simulink model "inverter_control"  (Simulink 8.5)
settings: Solver=ode23tb  StartTime=0.0  StopTime=0.1  RelTol=1e-4
values from neighbouring files (symbols this model uses):
  f_grid = 50    [inverter_settings.m]
  Kp = 2    [inverter_settings.m]
  L_f = 2e-3    (= 0.002)    [inverter_settings.m]
  R_f = 10e-3    (= 0.01)    [inverter_settings.m]
  Ti = 10e-3    (= 0.01)    [inverter_settings.m]
  V_dc = 700    [inverter_settings.m]
  V_grid = 230    [inverter_settings.m]
  wc = 1/0.05e-3    (= 20000)    [inverter_settings.m]
undefined symbols (not defined in the file or in its folder): j
libraries: powerlib x28, powerlib_meascontrol x3
settings Model: Creator=Pierre  LastModifiedBy=Pierre
settings DataIOCC: SignalLoggingSaveFormat=Dataset
settings OptimizationCC: ExpressionDepthLimit=128
settings DebuggingCC: UnderspecifiedInitializationDetection=Simplified  MergeDetectMultiDrivingBlocksExec=error  FcnCallInpInsideContextMsg=EnableAllAsError  StateNameClashWarn=none
settings GRTTargetCC: CombineOutputUpdateFcns=on  GRTInterface=off

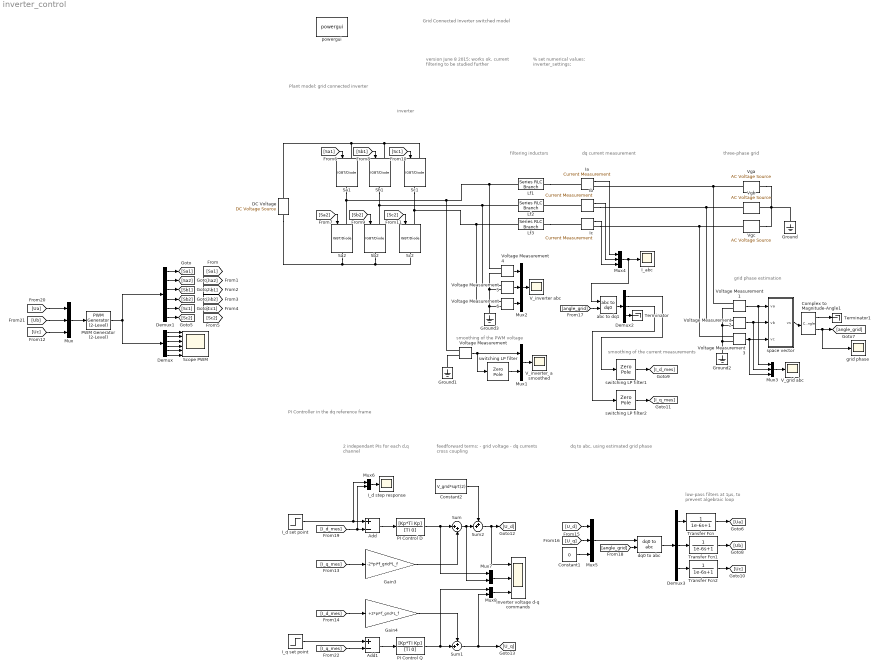
== system inverter_control ==
  note: smoothing of the current measurements
  note: feedforward terms:
      | - grid voltage
      | - dq currents cross coupling
  note: PI Controller
      | in the dq reference frame
  note: % set numerical values:
      | inverter_settings;
  note: version June 8 2015: works ok.
      | current filtering to be studied further
  note: Grid Connected Inverter
      | switched model
  note: 2 independant PIs
      | for each d,q channel
  note: dq to abc,
      | using estimated grid phase
  note: low-pass filters at 1µs,
      | to prevent algebraic loop
  note: inverter
  note: Plant model: grid connected inverter
  note: filtering inductors
  note: three-phase grid
  note: dq current measurement
  note: grid phase estimation
  note: smoothing of the PWM voltage
  Add : Sum  Inputs=+-
  Add1 : Sum  Inputs=+-
  Complex to Magnitude-Angle1 : ComplexToMagnitudeAngle
  Constant1 : Constant  Value=0
  Constant2 : Constant  Value=V_grid*sqrt(2)
  DC Voltage : powerlib/Electrical Sources/DC Voltage Source  Amplitude=V_dc  Measurements=None
  Demux : Demux  Outputs=6
  Demux1 : Demux  Outputs=6
  Demux2 : Demux  Outputs=3
  Demux3 : Demux  Outputs=3
  Gain3 : Gain  Gain=-2*pi*f_grid*L_f
  Gain4 : Gain  Gain=+2*pi*f_grid*L_f
  Ground{,1..3} (4 alike) : powerlib/Elements/Ground  LConnTagsString=a
  I_abc : Scope
      settings: TimeRange=2  YMin=0  YMax=12  SaveName=ScopeData4
  I_d set point : Step  Time=0.03  After=10  SampleTime=0
  I_d step response : Scope
      settings: TimeRange=2  YMin=-15  YMax=15  SaveName=ScopeData7
  I_q set point : Step  Time=0.01  After=0  SampleTime=0
  Ia : powerlib/Measurements/Current Measurement  PhasorSimulation=off  OutputType=Complex  PSBequivalent=0
  Ib : powerlib/Measurements/Current Measurement  PhasorSimulation=off  OutputType=Complex  PSBequivalent=0
  Ic : powerlib/Measurements/Current Measurement  PhasorSimulation=off  OutputType=Complex  PSBequivalent=0
  Inverter voltage d-q commands : Scope  NumInputPorts=3
      settings: TimeRange=2  YMin=0~-5~-5  YMax=12~5~5  SaveName=ScopeData6
  Lf1 : powerlib/Elements/Series RLC Branch  LConnTagsString=__new0  RConnTagsString=__new0  BranchType=RL  Resistance=R_f  Inductance=L_f  SetiL0=off  InitialCurrent=0  Capacitance=1e-6  Setx0=off  InitialVoltage=0  Measurements=None
  Lf2 : powerlib/Elements/Series RLC Branch  LConnTagsString=__new0  RConnTagsString=__new0  BranchType=RL  Resistance=R_f  Inductance=L_f  SetiL0=off  InitialCurrent=0  Capacitance=1e-6  Setx0=off  InitialVoltage=0  Measurements=None
  Lf3 : powerlib/Elements/Series RLC Branch  LConnTagsString=__new0  RConnTagsString=__new0  BranchType=RL  Resistance=R_f  Inductance=L_f  SetiL0=off  InitialCurrent=0  Capacitance=1e-6  Setx0=off  InitialVoltage=0  Measurements=None
  Mux{,2..5} (5 alike) : Mux  Inputs=3
  Mux{1,6..8} (4 alike) : Mux  Inputs=2
  PI Control D : TransferFcn  Numerator=[Kp*Ti Kp]  Denominator=[Ti 0]
  PI Control Q : TransferFcn  Numerator=[Kp*Ti Kp]  Denominator=[Ti 0]
  PWM Generator (2-Level) : powerlib_meascontrol/Pulse & Signal Generators/PWM Generator (2-Level)  ModulatorType=Three-phase bridge (6 pulses)  ModulatorMode=Unsynchronized  Fc=f_switch  Pc=90  nF=27  MinMax=[ -V_dc/2 V_dc/2 ]  SamplingTechnique=Symmetrical regular (single edge)  ModulatingSignals=off  m=0.8  Freq=60  Phase=0  Ts=0  ShowCarrierOutport=off
  Sa1 : powerlib/Power Electronics/IGBT//Diode  Ron=1e-3  Rs=1e5  Cs=inf  Measurements=off
  Sa2 : powerlib/Power Electronics/IGBT//Diode  Ron=1e-3  Rs=1e5  Cs=inf  Measurements=off
  Sb1 : powerlib/Power Electronics/IGBT//Diode  Ron=1e-3  Rs=1e5  Cs=inf  Measurements=off
  Sb2 : powerlib/Power Electronics/IGBT//Diode  Ron=1e-3  Rs=1e5  Cs=inf  Measurements=off
  Sc1 : powerlib/Power Electronics/IGBT//Diode  Ron=1e-3  Rs=1e5  Cs=inf  Measurements=off
  Sc2 : powerlib/Power Electronics/IGBT//Diode  Ron=1e-3  Rs=1e5  Cs=inf  Measurements=off
  Scope PWM : Scope  NumInputPorts=6
      settings: YMin=-5~-5~-5~-5~-5~-5  YMax=5~5~5~5~5~5
  Sum : Sum  Inputs=|++
  Sum1 : Sum  Inputs=++|
  Sum2 : Sum  Inputs=++|
  Terminator : Terminator
  Terminator1 : Terminator
  Transfer Fcn : TransferFcn  Denominator=[1e-6 1]
  Transfer Fcn1 : TransferFcn  Denominator=[1e-6 1]
  Transfer Fcn2 : TransferFcn  Denominator=[1e-6 1]
  V_grid abc : Scope
      settings: TimeRange=2  YMin=0  YMax=12  SaveName=ScopeData2
  V_inverter abc : Scope
      settings: TimeRange=2  YMin=0  YMax=12  SaveName=ScopeData5
  V_inverter_a smoothed : Scope
      settings: TimeRange=0.01780812410426348  YMin=-450  YMax=450
  Vga : powerlib/Electrical Sources/AC Voltage Source  Amplitude=V_grid*sqrt(2)  Phase=0  Frequency=f_grid  SampleTime=0  Measurements=None
  Vgb : powerlib/Electrical Sources/AC Voltage Source  Amplitude=V_grid*sqrt(2)  Phase=-120  Frequency=f_grid  SampleTime=0  Measurements=None
  Vgc : powerlib/Electrical Sources/AC Voltage Source  Amplitude=V_grid*sqrt(2)  Phase=-240  Frequency=f_grid  SampleTime=0  Measurements=None
  Voltage Measurement{,1..6} (7 alike) : powerlib/Measurements/Voltage Measurement  PhasorSimulation=off  OutputType=Complex  PSBequivalent=0
  abc to dq1 : powerlib_meascontrol/Transformations/abc to dq0  Alignment=Aligned with phase A axis
  dq0 to abc : powerlib_meascontrol/Transformations/dq0 to abc  Alignment=Aligned with phase A axis
  grid phase : Scope
      settings: TimeRange=2  YMin=0  YMax=12  SaveName=ScopeData3
  powergui : powerlib/powergui  Priority=1  SimulationMode=Continuous  SolverType=Tustin/Backward Euler (TBE)  SampleTime=50e-6  frequency=60  SPID=off  DisableSnubberDevices=on  DisableRonSwitches=on  DisableVfSwitches=on  SwTol=0  DisplayEquations=off  Interpol=off  methode=off  Ts=100  FunctionMessages=off  echomessages=off  HookPort=off  EnableUseOfTLC=off  x0status=blocks  frequencyindice=50  Pbase=100e6  ErrMax=1e-4  Iterations=50  UnitsV=kV  UnitsW=MW  buscounter=0  RestoreLinks=warning  ResistiveCurrentMeasurement=off  Frange=[0:2:500]  Ylog=off  Xlog=on  ShowGrid=off  save=off  variable=ZData  structure=0  ZoomFFT=off  StartTime=0.0  cycles=1  DisplayStyle=1  fundamental=60  FreqAxis=off  MaxFrequency=1000  frequencyindicesteady=1  RmsSteady=1  display=off
  space vector : Subsystem
  switching LP filter : ZeroPole  Zeros=[]  Poles=[-wc -wc -wc -wc]  Gain=[wc^4]
  switching LP filter1 : ZeroPole  Zeros=[]  Poles=[-wc -wc -wc]  Gain=[wc^3]
  switching LP filter2 : ZeroPole  Zeros=[]  Poles=[-wc -wc -wc]  Gain=[wc^3]
  wires:
  Mux/1 -> PWM Generator (2-Level)/1
  PWM Generator (2-Level)/1 -> Demux/1, Demux1/1
  Demux/1 -> Scope PWM/1
  Demux/3 -> Scope PWM/3
  Demux/4 -> Scope PWM/4
  Demux/5 -> Scope PWM/5
  Demux/6 -> Scope PWM/6
  Demux/2 -> Scope PWM/2
  Demux1/6 -> [Sc2]
  Demux1/1 -> [Sa1]
  Demux1/2 -> [Sa2]
  Demux1/3 -> [Sb1]
  Demux1/4 -> [Sb2]
  Demux1/5 -> [Sc1]
  [Sa1] -> Sa1/1
  [Sa2] -> Sa2/1
  [Sb1] -> Sb1/1
  [Sc1] -> Sc1/1
  [Sc2] -> Sc2/1
  [Sb2] -> Sb2/1
  Mux1/1 -> V_inverter_a smoothed/1
  switching LP filter/1 -> Mux1/2
  Mux2/1 -> V_inverter abc/1
  Voltage Measurement1/1 -> Mux3/1, space vector/1(va)
  Voltage Measurement2/1 -> Mux3/2, space vector/2(vb)
  Voltage Measurement3/1 -> space vector/3(vc), Mux3/3
  space vector/1(vs) -> Complex to Magnitude-Angle1/1
  Mux3/1 -> V_grid abc/1
  Mux4/1 -> I_abc/1, abc to dq1/1
  Ia/1 -> Mux4/1
  Ib/1 -> Mux4/2
  Ic/1 -> Mux4/3
  Voltage Measurement4/1 -> Mux2/1
  Voltage Measurement5/1 -> Mux2/2
  Voltage Measurement6/1 -> Mux2/3
  Complex to Magnitude-Angle1/2 -> [angle_grid], grid phase/1
  [angle_grid] -> abc to dq1/2
  Demux2/3 -> Terminator/1
  [angle_grid] -> dq0 to abc/2
  [I_d_mes] -> Mux6/2, Add/2
  I_d set point/1 -> Mux6/1, Add/1
  Add/1 -> PI Control D/1
  Mux5/1 -> dq0 to abc/1
  Demux3/1 -> Transfer Fcn/1
  [I_q_mes] -> Add1/2
  I_q set point/1 -> Add1/1
  Add1/1 -> PI Control Q/1
  Complex to Magnitude-Angle1/1 -> Terminator1/1
  Demux3/2 -> Transfer Fcn1/1
  Demux3/3 -> Transfer Fcn2/1
  Gain4/1 -> Sum1/1
  PI Control Q/1 -> Mux8/1, Sum1/2
  dq0 to abc/1 -> Demux3/1
  Sum/1 -> Mux7/2, Sum2/2
  Mux6/1 -> I_d step response/1
  Sum2/1 -> Inverter voltage d-q commands/1, [U_d]
  Sum1/1 -> Mux8/2, [U_q]
  Gain3/1 -> Sum/2
  PI Control D/1 -> Mux7/1, Sum/1
  [U_d] -> Mux5/1
  [U_q] -> Mux5/2
  Constant1/1 -> Mux5/3
  Mux7/1 -> Inverter voltage d-q commands/2
  Mux8/1 -> Inverter voltage d-q commands/3
  Transfer Fcn/1 -> [Ua]
  Transfer Fcn1/1 -> [Ub]
  Transfer Fcn2/1 -> [Uc]
  [I_q_mes] -> Gain3/1
  [I_d_mes] -> Gain4/1
  Constant2/1 -> Sum2/1
  [Uc] -> Mux/3
  [Ub] -> Mux/2
  [Ua] -> Mux/1
  abc to dq1/1 -> Demux2/1
  switching LP filter1/1 -> [I_d_mes]
  switching LP filter2/1 -> [I_q_mes]
  Demux2/1 -> switching LP filter1/1
  Demux2/2 -> switching LP filter2/1
  Voltage Measurement/1 -> switching LP filter/1, Mux1/1
  connections:
  Ground1/LConn1 -- Voltage Measurement/LConn2
  Sa2/RConn1 -- DC Voltage/LConn1 -- Sb2/RConn1 -- Sc2/RConn1
  Sa1/LConn1 -- DC Voltage/RConn1 -- Sb1/LConn1 -- Sc1/LConn1
  Voltage Measurement2/LConn1 -- Vgb/RConn1 -- Ib/RConn1
  Voltage Measurement3/LConn1 -- Vgc/RConn1 -- Ic/RConn1
  Voltage Measurement1/LConn1 -- Vga/RConn1 -- Ia/RConn1
  Lf1/LConn1 -- Voltage Measurement/LConn1 -- Sa2/LConn1 -- Sa1/RConn1 -- Voltage Measurement4/LConn1
  Voltage Measurement1/LConn2 -- Voltage Measurement2/LConn2 -- Voltage Measurement3/LConn2 -- Ground2/LConn1
  Voltage Measurement6/LConn1 -- Sc1/RConn1 -- Sc2/LConn1 -- Lf3/LConn1
  Voltage Measurement5/LConn1 -- Sb2/LConn1 -- Sb1/RConn1 -- Lf2/LConn1
  Voltage Measurement4/LConn2 -- Voltage Measurement5/LConn2 -- Voltage Measurement6/LConn2 -- Ground3/LConn1
  Ground/LConn1 -- Vgc/LConn1 -- Vga/LConn1 -- Vgb/LConn1
  Lf3/RConn1 -- Ic/LConn1
  Lf1/RConn1 -- Ia/LConn1
  Ib/LConn1 -- Lf2/RConn1

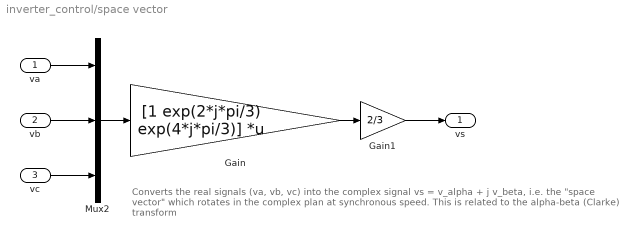
== system inverter_control/space vector ==
  note: Converts the real signals (va, vb, vc)
      | into the complex signal vs = v_alpha + j v_beta, i.e. the "space vector" which rotates in the complex plan at synchronous speed.
      | This is related to the alpha-beta (Clarke) transform
  va : Inport
  vb : Inport  Port=2
  vc : Inport  Port=3
  Gain : Gain  Gain=[1 exp(2*j*pi/3) exp(4*j*pi/3)]  Multiplication=Matrix(K*u) (u vector)
  Gain1 : Gain  Gain=2/3
  Mux2 : Mux  Inputs=3
  vs : Outport
  wires:
  Mux2/1 -> Gain/1
  vb/1 -> Mux2/2
  Gain1/1 -> vs/1
  va/1 -> Mux2/1
  Gain/1 -> Gain1/1
  vc/1 -> Mux2/3
